simulink model "walk1"  (R2020a)
settings: Solver=FixedStepDiscrete  StartTime=0.0  StopTime=15  FixedStep=deltaT  RelTol=1e-3
InitFcn:
  | %****NOTE: you must change the line below
  | % to the IP address for YOUR ROS master!****
  | deltaT = 0.1;
  | ipaddress = 'http://10.4.155.40:11311';
  | 
  | % --- Start MATLAB Global Node
  | try % try to print list of ROS nodes
  |     rosnode list
  |     clc
  | % if error from rosnode list,
  | % initialize ROS global node from MATLAB
  | catch exp
  |     rosinit(ipaddress)  % only if error: rosinit
  |     pause(5)
  | end
StartFcn:
  | % Publishers to ROS topics for left, right
  | % upper arm joint commands
  | Larm = rospublisher('/darwin/j_high_arm_l_position_controller/command','std_msgs/Float64');
  | Rarm = rospublisher('/darwin/j_high_arm_r_position_controller/command','std_msgs/Float64');
  | 
  | % Create ROS messages to publishers
  | Ldown = rosmessage(Larm);
  | Rdown = rosmessage(Rarm);
  | Ldown2 = rosmessage(Larm);
  | Rdown2 = rosmessage(Rarm);
  | 
  | % move upper arm joint to 0.5 radian
  | Ldown.Data = 0.5;
  | Rdown.Data = 0.5;
  | 
  | % move upper arm joint to 0.8 radian
  | Ldown2.Data = 0.8;
  | Rdown2.Data = 0.8;
  | 
  | % move arms to 0.5 radian during two-second period,
  | % then to 0.8 radian during another
  | % two-second period (arms move synchronously)
  | send(Larm,Ldown);
  | send(Rarm,Rdown);
  | pause(2)
  | send(Larm,Ldown2);
  | send(Rarm,Rdown2);
  | pause(2)
  | 
  | disturb = rossvcclient('/gazebo/apply_body_wrench');
  | disturbmsg = rosmessage(disturb);
  | disturbmsg.ReferenceFrame = 'world';
  | disturbmsg.ReferencePoint.X = 0; disturbmsg.ReferencePoint.Y = 0; disturbmsg.ReferencePoint.Z = 0;
  | disturbmsg.Wrench.Force.X = 0.0; disturbmsg.Wrench.Force.Y = 0.0; disturbmsg.Wrench.Force.Z = 0.0;
  | disturbmsg.Wrench.Torque.X = 0.0; disturbmsg.Wrench.Torque.Y = 0.0; disturbmsg.Wrench.Torque.Z = 0.0;
  | disturbmsg.StartTime.Sec = 0; disturbmsg.StartTime.Nsec = 0;
  | disturbmsg.Duration.Sec = 0; disturbmsg.Duration.Nsec = 500000000;
StopFcn:
  | rosshutdown
model workspace (MAT data in the model file):
  SL_ROS_VariableLengthArrays_MaxSizes.CommonInfo.ArrayTruncateAction = 'EmitWarning'
  SL_ROS_VariableLengthArrays_MaxSizes.MsgTypeMap = containers.Map
  SL_ROS_VariableLengthArrays_MaxSizes.MsgTypeMap.serialization.keys = {'gazebo_msgs/ApplyBodyWrenchRequest', 'sensor_msgs/JointState'}
  SL_ROS_VariableLengthArrays_MaxSizes.MsgTypeMap.serialization.values{1}(1).PropertyName = 'BodyName'
  SL_ROS_VariableLengthArrays_MaxSizes.MsgTypeMap.serialization.values{1}(1).DataType = 'uint8'
  SL_ROS_VariableLengthArrays_MaxSizes.MsgTypeMap.serialization.values{1}(1).MaxLength = 19
  SL_ROS_VariableLengthArrays_MaxSizes.MsgTypeMap.serialization.values{1}(2).PropertyName = 'ReferenceFrame'
  SL_ROS_VariableLengthArrays_MaxSizes.MsgTypeMap.serialization.values{1}(2).DataType = 'uint8'
  SL_ROS_VariableLengthArrays_MaxSizes.MsgTypeMap.serialization.values{1}(2).MaxLength = 5
  SL_ROS_VariableLengthArrays_MaxSizes.MsgTypeMap.serialization.values{2}(1).PropertyName = 'Effort'
  SL_ROS_VariableLengthArrays_MaxSizes.MsgTypeMap.serialization.values{2}(1).DataType = 'double'
  SL_ROS_VariableLengthArrays_MaxSizes.MsgTypeMap.serialization.values{2}(1).MaxLength = 128
  SL_ROS_VariableLengthArrays_MaxSizes.MsgTypeMap.serialization.values{2}(2).PropertyName = 'Name'
  SL_ROS_VariableLengthArrays_MaxSizes.MsgTypeMap.serialization.values{2}(2).DataType = 'std_msgs/String'
  SL_ROS_VariableLengthArrays_MaxSizes.MsgTypeMap.serialization.values{2}(2).MaxLength = 24
  SL_ROS_VariableLengthArrays_MaxSizes.MsgTypeMap.serialization.values{2}(3).PropertyName = 'Position'
  SL_ROS_VariableLengthArrays_MaxSizes.MsgTypeMap.serialization.values{2}(3).DataType = 'double'
  SL_ROS_VariableLengthArrays_MaxSizes.MsgTypeMap.serialization.values{2}(3).MaxLength = 128
  SL_ROS_VariableLengthArrays_MaxSizes.MsgTypeMap.serialization.values{2}(4).PropertyName = 'Velocity'
  SL_ROS_VariableLengthArrays_MaxSizes.MsgTypeMap.serialization.values{2}(4).DataType = 'double'
  SL_ROS_VariableLengthArrays_MaxSizes.MsgTypeMap.serialization.values{2}(4).MaxLength = 128
  SL_ROS_VariableLengthArrays_MaxSizes.MsgTypeMap.serialization.uniformity = 0
  SL_ROS_VariableLengthArrays_MaxSizes.MsgTypeMap.serialization.keyType = 'char'
  SL_ROS_VariableLengthArrays_MaxSizes.MsgTypeMap.serialization.valueType = 'any'
undefined symbols (not defined in the file or in its folder): Linear
libraries: robotlib x13, realtime_pacer_lib x1
settings Model: Creator=JerryLee  LastModifiedBy=JerryLee
settings OptimizationCC: EnhancedBackFolding=on  PassReuseOutputArgsAs=Individual arguments  ZeroExternalMemoryAtStartup=off  ZeroInternalMemoryAtStartup=off  MaxStackSize=64  OptimizeBlockOrder=speed  DifferentSizesBufferReuse=on  OptimizationCustomize=off  EfficientTunableParamExpr=on
settings DebuggingCC: ParameterTunabilityLossMsg=error
settings HardwareCC: ProdBitPerPointer=32  ProdBitPerSizeT=32  ProdBitPerPtrDiffT=32  ProdLargestAtomicFloat=None  ProdIntDivRoundTo=Undefined  ProdEndianess=Unspecified  ProdWordSize=32  ProdHWDeviceType=Generic->Unspecified (assume 32-bit Generic)  UseEmbeddedCoderFeatures=off
settings SFSimCC: MATLABDynamicMemAlloc=off
settings RTWCC: SystemTargetFile=ert.tlc  HardwareBoard=Robot Operating System (ROS)  TemplateMakefile=ert_default_tmf  Toolchain=Catkin  TargetLang=C++
settings CodeAppCC: ForceParamTrailComments=on  IgnoreCustomStorageClasses=off  OperatorAnnotations=on  SimulinkDataObjDesc=on  SFDataObjDesc=on  InsertBlockDesc=on
settings ERTTargetCC: SupportNonInlinedSFcns=on

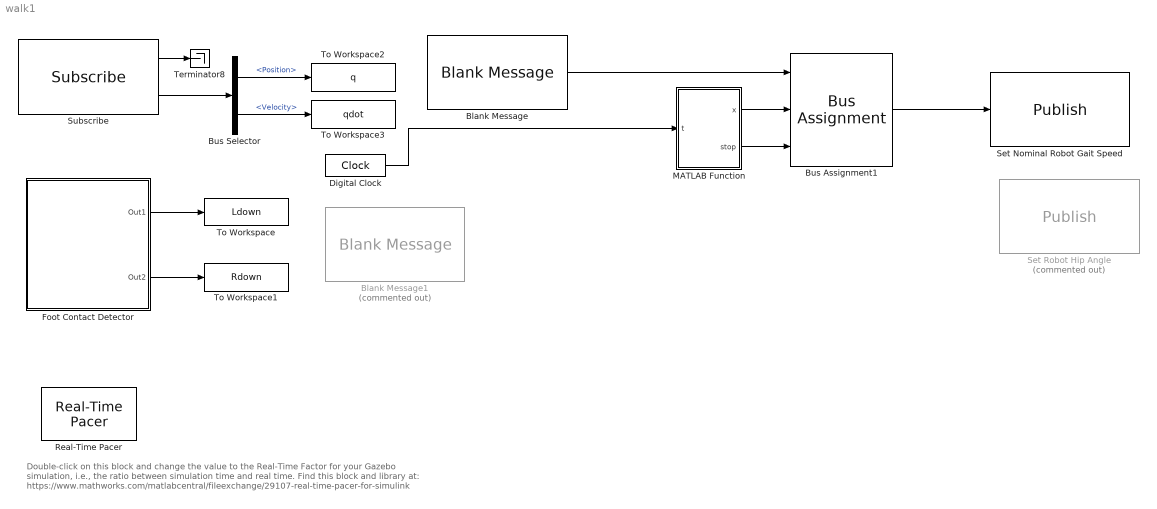
== system walk1 ==
  note: Double-click on this block and
      | change the value to the Real-Time
      | Factor for your Gazebo simulation,
      | i.e., the ratio between simulation time
      | and real time.
      |
      | Find this block and library at:
      | https://www.mathworks.com/matlabcentral/fileexchange/29107-real-time-pacer-for-simulink
  Blank Message : robotlib/Blank Message  messageClass=Message  entityType=geometry_msgs/Twist  messageType=geometry_msgs/Twist  SampleTime=deltaT
  Blank Message1 : robotlib/Blank Message  Commented=on  messageClass=Message  entityType=std_msgs/Float64  messageType=std_msgs/Float64  SampleTime=deltaT
  Bus Assignment1 : BusAssignment  AssignedSignals=Linear.X,Linear.Z
  Bus Selector : BusSelector  OutputSignals=Position,Velocity
  Digital Clock : DigitalClock  SampleTime=deltaT
  Foot Contact Detector : Subsystem
  MATLAB Function : MATLAB Function  TreatAsAtomicUnit=on
  Real-Time Pacer : realtime_pacer_lib/Real-Time Pacer  simTimePerRealTime=0.5
      settings: SourceProductName=Real-Time Pacer
  Set Nominal Robot Gait Speed : robotlib/Publish  topicSource=Select from ROS network  topic=/darwin/cmd_vel  messageType=geometry_msgs/Twist  messageQueueLength=1
  Set Robot Hip Angle : robotlib/Publish  Commented=on  topicSource=Select from ROS network  topic=/darwin/j_thigh2_r_position_controller/command  messageType=std_msgs/Float64  messageQueueLength=1
  Subscribe : robotlib/Subscribe  topicSource=Select from ROS network  topic=/darwin/joint_states  messageType=sensor_msgs/JointState  sampleTime=deltaT  messageQueueLength=1
  Terminator8 : Terminator
  To Workspace : ToWorkspace  VariableName=Ldown  SampleTime=deltaT
  To Workspace1 : ToWorkspace  VariableName=Rdown  SampleTime=deltaT
  To Workspace2 : ToWorkspace  VariableName=q  SampleTime=deltaT
  To Workspace3 : ToWorkspace  VariableName=qdot  SampleTime=deltaT
  wires:
  Subscribe/1 -> Terminator8/1
  Foot Contact Detector/2(Out2) -> To Workspace1/1
  Foot Contact Detector/1(Out1) -> To Workspace/1
  Subscribe/2 -> Bus Selector/1
  Bus Selector/1 -> To Workspace2/1  "<Position>"
  Bus Selector/2 -> To Workspace3/1  "<Velocity>"
  Blank Message/1 -> Bus Assignment1/1
  MATLAB Function/1(x) -> Bus Assignment1/2
  Digital Clock/1 -> MATLAB Function/1(t)
  Bus Assignment1/1 -> Set Nominal Robot Gait Speed/1
  MATLAB Function/2(stop) -> Bus Assignment1/3

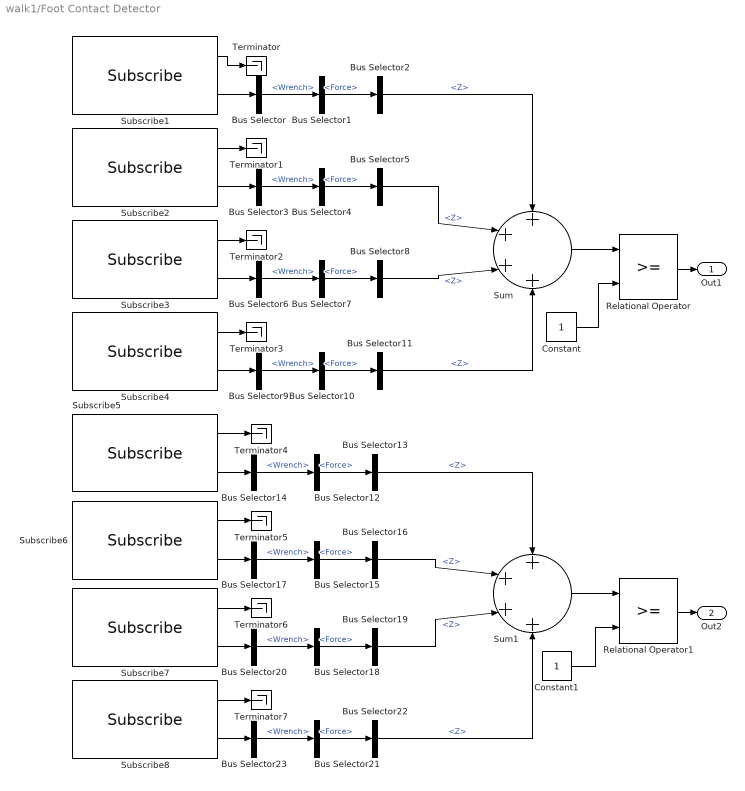
== system walk1/Foot Contact Detector ==
  Bus Selector{,3,6,9,14,17,20,23} (8 alike) : BusSelector  OutputSignals=Wrench
  Bus Selector{1,4,7,10,12,15,18,21} (8 alike) : BusSelector  OutputSignals=Force
  Bus Selector{2,5,8,11,13,16,19,22} (8 alike) : BusSelector  OutputSignals=Z
  Constant : Constant
  Constant1 : Constant
  Relational Operator : RelationalOperator  OutDataTypeStr=boolean  RndMeth=Simplest
  Relational Operator1 : RelationalOperator  OutDataTypeStr=boolean  RndMeth=Simplest
  Subscribe1 : robotlib/Subscribe  topicSource=Select from ROS network  topic=/leap_one/left_foot_sensor_m0  messageType=geometry_msgs/WrenchStamped  sampleTime=deltaT  messageQueueLength=1
  Subscribe2 : robotlib/Subscribe  topicSource=Select from ROS network  topic=/leap_one/left_foot_sensor_m1  messageType=geometry_msgs/WrenchStamped  sampleTime=deltaT  messageQueueLength=1
  Subscribe3 : robotlib/Subscribe  topicSource=Select from ROS network  topic=/leap_one/left_foot_sensor_m2  messageType=geometry_msgs/WrenchStamped  sampleTime=deltaT  messageQueueLength=1
  Subscribe4 : robotlib/Subscribe  topicSource=Select from ROS network  topic=/leap_one/left_foot_sensor_m3  messageType=geometry_msgs/WrenchStamped  sampleTime=deltaT  messageQueueLength=1
  Subscribe5 : robotlib/Subscribe  topicSource=Select from ROS network  topic=/leap_one/right_foot_sensor_m0  messageType=geometry_msgs/WrenchStamped  sampleTime=deltaT  messageQueueLength=1
  Subscribe6 : robotlib/Subscribe  topicSource=Select from ROS network  topic=/leap_one/right_foot_sensor_m1  messageType=geometry_msgs/WrenchStamped  sampleTime=deltaT  messageQueueLength=1
  Subscribe7 : robotlib/Subscribe  topicSource=Select from ROS network  topic=/leap_one/right_foot_sensor_m2  messageType=geometry_msgs/WrenchStamped  sampleTime=deltaT  messageQueueLength=1
  Subscribe8 : robotlib/Subscribe  topicSource=Select from ROS network  topic=/leap_one/right_foot_sensor_m3  messageType=geometry_msgs/WrenchStamped  sampleTime=deltaT  messageQueueLength=1
  Sum : Sum  Inputs=4
  Sum1 : Sum  Inputs=4
  Terminator{,1..7} (8 alike) : Terminator
  Out1 : Outport
  Out2 : Outport  Port=2
  wires:
  Bus Selector6/1 -> Bus Selector7/1  "<Wrench>"
  Subscribe8/2 -> Bus Selector23/1
  Bus Selector22/1 -> Sum1/4  "<Z>"
  Bus Selector8/1 -> Sum/3  "<Z>"
  Subscribe5/1 -> Terminator4/1
  Bus Selector/1 -> Bus Selector1/1  "<Wrench>"
  Subscribe1/2 -> Bus Selector/1
  Bus Selector2/1 -> Sum/1  "<Z>"
  Bus Selector20/1 -> Bus Selector18/1  "<Wrench>"
  Bus Selector19/1 -> Sum1/3  "<Z>"
  Subscribe2/2 -> Bus Selector3/1
  Bus Selector17/1 -> Bus Selector15/1  "<Wrench>"
  Constant/1 -> Relational Operator/2
  Bus Selector3/1 -> Bus Selector4/1  "<Wrench>"
  Relational Operator1/1 -> Out2/1
  Bus Selector18/1 -> Bus Selector19/1  "<Force>"
  Bus Selector9/1 -> Bus Selector10/1  "<Wrench>"
  Subscribe2/1 -> Terminator1/1
  Bus Selector4/1 -> Bus Selector5/1  "<Force>"
  Bus Selector16/1 -> Sum1/2  "<Z>"
  Subscribe7/1 -> Terminator6/1
  Relational Operator/1 -> Out1/1
  Bus Selector13/1 -> Sum1/1  "<Z>"
  Constant1/1 -> Relational Operator1/2
  Subscribe7/2 -> Bus Selector20/1
  Bus Selector23/1 -> Bus Selector21/1  "<Wrench>"
  Subscribe6/2 -> Bus Selector17/1
  Subscribe6/1 -> Terminator5/1
  Bus Selector10/1 -> Bus Selector11/1  "<Force>"
  Bus Selector21/1 -> Bus Selector22/1  "<Force>"
  Sum/1 -> Relational Operator/1
  Subscribe3/1 -> Terminator2/1
  Bus Selector11/1 -> Sum/4  "<Z>"
  Bus Selector5/1 -> Sum/2  "<Z>"
  Subscribe4/2 -> Bus Selector9/1
  Subscribe5/2 -> Bus Selector14/1
  Subscribe3/2 -> Bus Selector6/1
  Bus Selector7/1 -> Bus Selector8/1  "<Force>"
  Subscribe1/1 -> Terminator/1
  Sum1/1 -> Relational Operator1/1
  Bus Selector15/1 -> Bus Selector16/1  "<Force>"
  Bus Selector1/1 -> Bus Selector2/1  "<Force>"
  Subscribe4/1 -> Terminator3/1
  Bus Selector14/1 -> Bus Selector12/1  "<Wrench>"
  Subscribe8/1 -> Terminator7/1
  Bus Selector12/1 -> Bus Selector13/1  "<Force>"

== matlab function walk1/MATLAB Function ==
  data: x output; t input; stop output
function [x,stop] = fcn(t)

% % forward walk:
% fore.Linear.X = 1; fore.Linear.Y = 0; fore.Linear.Z = 0; 
% fore.Angular.X = 0; fore.Angular.Y = 0; fore.Angular.Z = 0;
% 
% % backward walk:
% back.Linear.X = -1; back.Linear.Y = 0; back.Linear.Z = 0; 
% back.Angular.X = 0; back.Angular.Y = 0; back.Angular.Z = 0;
% 
% % come to stop:
% stop.Linear.X = 0; stop.Linear.Y = 0; stop.Linear.Z = 0; 
% stop.Angular.X = 0; stop.Angular.Y = 0; stop.Angular.Z = 0;

if t < 10
    x = 1;
else
    x = 0;
end

if t > 5 && t < 8
    stop = 0; % change this to 10 to stop these commands to robot
else
    stop = 0;
end
